simulink model "SolarMicroGrid"  (R2024b)
settings: Solver=VariableStepAuto  StartTime=0.0  StopTime=1  RelTol=1e-3
libraries: spsSeriesRLCBranchLib x9, spsMosfetLib x4, spsGroundLib x1, spsTriangleGeneratorLib x1, spsPVArrayLib x1, spsVoltageMeasurementLib x1, spsLinearTransformerLib x1, sps_lib x1
settings Model: Creator=Zidane Hadeed  LastModifiedBy=Zidane Hadeed

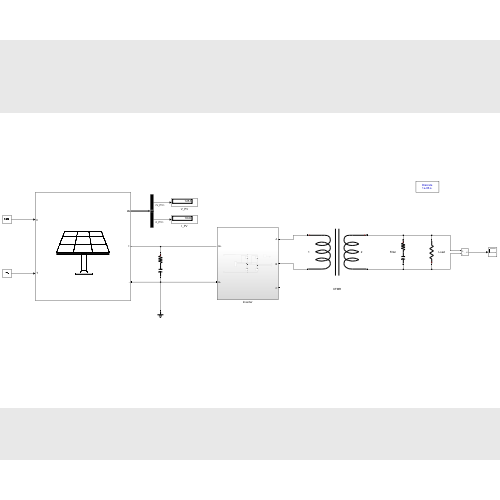
[thumbnail: Simulink's stored preview of the top-level diagram]
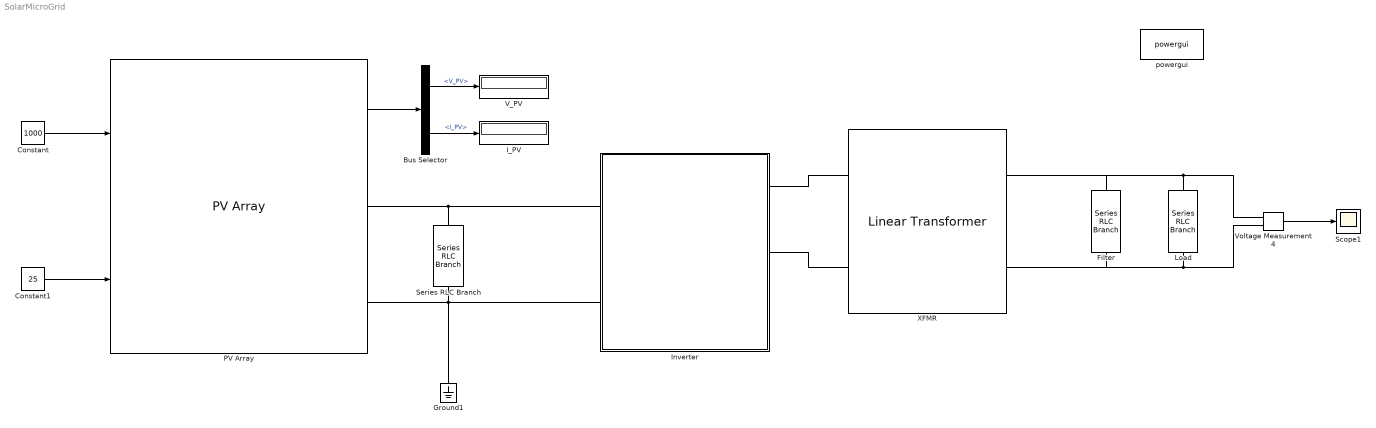
== system SolarMicroGrid ==
  Bus Selector : BusSelector  OutputSignals=V_PV,I_PV
  Constant : Constant  Value=1000
  Constant1 : Constant  Value=25
  Filter : spsSeriesRLCBranchLib/Series RLC Branch  LConnTagsString=__new0  RConnTagsString=__new0  BranchType=RC  Resistance=1e-3  Inductance=1e-3  SetiL0=off  InitialCurrent=0  Capacitance=1e-6  Setx0=off  InitialVoltage=0  Measurements=None
  Ground1 : spsGroundLib/Ground  LConnTagsString=a
  I_PV : Display
  Inverter : Subsystem
  Load : spsSeriesRLCBranchLib/Series RLC Branch  LConnTagsString=__new0  RConnTagsString=__new0  BranchType=R  Resistance=10e3  Inductance=1e-3  SetiL0=off  InitialCurrent=0  Capacitance=1e-6  Setx0=off  InitialVoltage=0  Measurements=None
  PV Array : spsPVArrayLib/PV Array  Npar=4  Nser=3  PlotType=array @ 25 deg.C & specified irradiances  S_vec="[ 1000  800  500 ]"  Temp_C_vec="[ 45 25  ]"  ModuleName=Aavid Solar ASMS-165P  PlotWhenSelected=off  Pm=164.85  Ncell=72  Voc=43.5  Isc=5.25  Vm=35  Im=4.71  beta_Voc_pc=-0.393  alpha_Isc_pc=0.03  beta_Voc=-0.17095  alpha_Isc=0.001575  IL=5.2764  I0=4.9875e-10  nI=1.0218  Rsh=125.0069  Rs=0.62818  RobustModel=off  RobustCellTemperature=313.3991  BAL=on  Tc=1e-6  Tfilter=5e-5
  Scope1 : Scope
  Series RLC Branch : spsSeriesRLCBranchLib/Series RLC Branch  LConnTagsString=__new0  RConnTagsString=__new0  BranchType=RC  Resistance=1e-2  Inductance=1e-3  SetiL0=off  InitialCurrent=0  Capacitance=4700e-6  Setx0=off  InitialVoltage=0  Measurements=None
  V_PV : Display
  Voltage Measurement4 : spsVoltageMeasurementLib/Voltage Measurement  PhasorSimulation=off  OutputType=Complex  PSBequivalent=0
  XFMR : spsLinearTransformerLib/Linear Transformer  UNITS=SI  NominalPower=[ 5e3 60 ]  winding1=[120 4.3218 0.45856]  winding2=[240 17.2872 1.83424]  ThreeWindings=off  winding3=[3.15e+05 0.7938 0.084225]  RmLm=[1.0804e+06 2866]  Measurements=All voltages and currents  DataType=on
  powergui : sps_lib/powergui  Priority=1  SimulationMode=Discrete  SampleTime=1e-6  frequency=60  Iterations=50  frequencyindice=0  Pbase=100e6  ErrMax=1e-4  UnitsV=kV  UnitsW=MW  buscounter=0  FunctionMessages=off  echomessages=off  EnableUseOfTLC=off  CurrentSourceSwitches=off  DisableSnubberDevices=off  DisableRonSwitches=off  DisableVfSwitches=off  DisplayEquations=off  AutomaticDiscreteSolvers=off  SolverType=Tustin/Backward Euler (TBE)  Interpol=off  ExternalGateDelay=off  methode=off  Ts=100  x0status=blocks  SPID=on  SwTol=0  HookPort=off  NonlinearTolerance=1e-4  nMaxIteration=100  ContinueOnMaxIteration=off  RestoreLinks=warning  ResistiveCurrentMeasurement=off  Frange=[0:2:500]  Ylog=off  Xlog=on  ShowGrid=off  save=off  variable=ZData  structure=0  ZoomFFT=off  StartTime=0.0  cycles=1  DisplayStyle=1  fundamental=60  FreqAxis=off  MaxFrequency=1000  frequencyindicesteady=1  RmsSteady=1  display=off
  wires:
  Voltage Measurement4/1 -> Scope1/1
  Constant1/1 -> PV Array/2
  PV Array/1 -> Bus Selector/1
  Constant/1 -> PV Array/1
  Bus Selector/1 -> V_PV/1  "<V_PV>"
  Bus Selector/2 -> I_PV/1  "<I_PV>"
  connections:
  Series RLC Branch/LConn1 -- Inverter/LConn1 -- PV Array/RConn1
  PV Array/RConn2 -- Ground1/LConn1 -- Series RLC Branch/RConn1 -- Inverter/LConn2
  Voltage Measurement4/LConn1 -- XFMR/RConn1 -- Filter/LConn1 -- Load/RConn1
  Load/LConn1 -- Filter/RConn1 -- XFMR/RConn2 -- Voltage Measurement4/LConn2
  XFMR/LConn1 -- Inverter/RConn1
  Inverter/RConn2 -- XFMR/LConn2

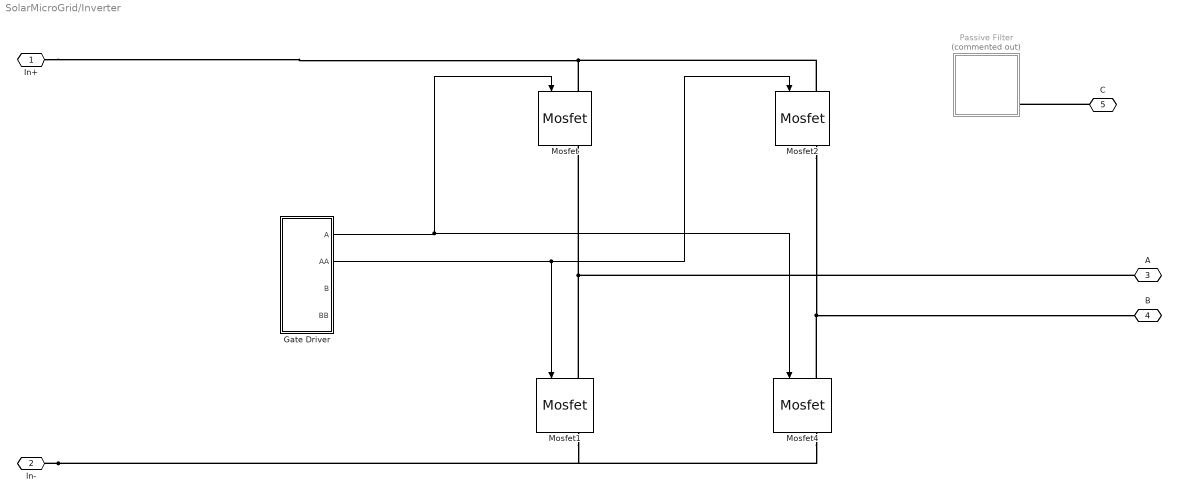
== system SolarMicroGrid/Inverter ==
  Gate Driver : Subsystem
  Mosfet{,1..2,4} (4 alike) : spsMosfetLib/Mosfet  Ron=0.1  Lon=0  Rd=0.01  Vfd=0  IC=0  Rs=1e5  Cs=inf  Measurements=on
  Passive Filter : Subsystem  Commented=on
      settings: PortSchema="{\"entries\":[{\"content\":{\"sides\":[{\"content\":{\"connectorIds\":[\"LConn1\",\"LConn2\",\"LConn3\"]},\"type\":\"ConnectorPlacement.EquallySpacedRectSide\",\"uuid\":\"62e55c9e-b411-4f10-a29f-aa0c5be36897\"},{\"content\":{\"connectorIds\":[\"RConn1\",\"RConn2\",\"RConn3\"],\"side\":\"RIGHT\"},\"type\":\"ConnectorPlacement.EquallySpacedRectSide\",\"uuid\":\"476f1a27-74f2-436a-8fc3-e2e5d83bb21b\"},{\"content\":{\"side\":\"TOP\"},\"type\":\"ConnectorPlacement.EquallySpacedRectSide\",\"uuid\":\"6a538d83-3a6b-4d9f-b9e9-43834189a8fd\"},{\"content\":{\"connectorIds\":[\"RConn4\"],\"side\":\"BOTTOM\"},\"type\":\"ConnectorPlacement.EquallySpacedRectSide\",\"uuid\":\"d798d2e6-cd10-429f-9f9b-8383104bce78\"}]},\"type\":\"ConnectorPlacement.EquallySpacedConnector\",\"uuid\":\"0b9f9509-cccf-4838-84a5-b9f3e67ee63a\"}],\"packageUris\":[\"http://schema.mathworks.com/mf0/Connector/R2020b\"],\"version\":\"1.0\"}"
  In+ : PMIOPort  Side=Left
  In- : PMIOPort  Port=2  Side=Left
  A : PMIOPort  Port=3  Side=Right
  B : PMIOPort  Port=4  Side=Right
  C : PMIOPort  Port=5  Side=Right
  wires:
  Gate Driver/1(A) -> Mosfet4/1, Mosfet/1
  Gate Driver/2(AA) -> Mosfet2/1, Mosfet1/1
  connections:
  In-/RConn1 -- Mosfet4/RConn1 -- Mosfet1/RConn1
  In+/RConn1 -- Mosfet2/LConn1 -- Mosfet/LConn1
  Mosfet1/LConn1 -- A/RConn1 -- Mosfet/RConn1
  Mosfet2/RConn1 -- Mosfet4/LConn1 -- B/RConn1
  C/RConn1 -- Passive Filter/RConn3

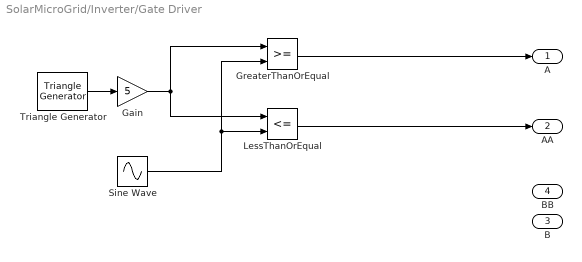
== system SolarMicroGrid/Inverter/Gate Driver ==
  Gain : Gain  Gain=5
  GreaterThanOrEqual : RelationalOperator  OutDataTypeStr=boolean  RndMeth=Simplest  InputSameDT=off
  LessThanOrEqual : RelationalOperator  Operator=<=  OutDataTypeStr=boolean  RndMeth=Simplest  InputSameDT=off
  Sine Wave : Sin  Amplitude=5  Frequency=100*pi  SampleTime=0
  Triangle Generator : spsTriangleGeneratorLib/Triangle Generator  Freq=300  Phase=0  Ts=0
  A : Outport
  AA : Outport  Port=2
  B : Outport  Port=3
  BB : Outport  Port=4
  wires:
  Sine Wave/1 -> GreaterThanOrEqual/2, LessThanOrEqual/2
  Triangle Generator/1 -> Gain/1
  Gain/1 -> LessThanOrEqual/1, GreaterThanOrEqual/1
  GreaterThanOrEqual/1 -> A/1
  LessThanOrEqual/1 -> AA/1

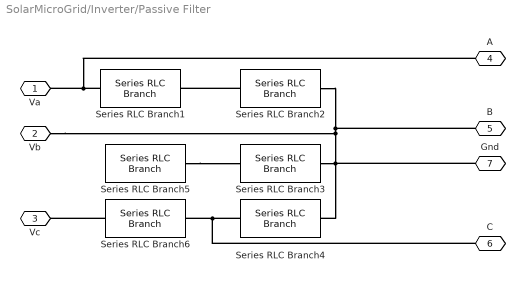
== system SolarMicroGrid/Inverter/Passive Filter ==
  Series RLC Branch1 : spsSeriesRLCBranchLib/Series RLC Branch  LConnTagsString=__new0  RConnTagsString=__new0  BranchType=L  Resistance=1  Inductance=100e-3  SetiL0=off  InitialCurrent=0  Capacitance=540e-3  Setx0=off  InitialVoltage=0  Measurements=None
  Series RLC Branch2 : spsSeriesRLCBranchLib/Series RLC Branch  LConnTagsString=__new0  RConnTagsString=__new0  BranchType=C  Resistance=1  Inductance=1e-3  SetiL0=off  InitialCurrent=0  Capacitance=0.1e-6  Setx0=off  InitialVoltage=0  Measurements=None
  Series RLC Branch3 : spsSeriesRLCBranchLib/Series RLC Branch  LConnTagsString=__new0  RConnTagsString=__new0  BranchType=C  Resistance=1  Inductance=1e-3  SetiL0=off  InitialCurrent=0  Capacitance=100e-6  Setx0=off  InitialVoltage=0  Measurements=None
  Series RLC Branch4 : spsSeriesRLCBranchLib/Series RLC Branch  LConnTagsString=__new0  RConnTagsString=__new0  BranchType=C  Resistance=1  Inductance=1e-3  SetiL0=off  InitialCurrent=0  Capacitance=100e-6  Setx0=off  InitialVoltage=0  Measurements=None
  Series RLC Branch5 : spsSeriesRLCBranchLib/Series RLC Branch  LConnTagsString=__new0  RConnTagsString=__new0  BranchType=L  Resistance=1  Inductance=100e-3  SetiL0=off  InitialCurrent=0  Capacitance=540e-3  Setx0=off  InitialVoltage=0  Measurements=None
  Series RLC Branch6 : spsSeriesRLCBranchLib/Series RLC Branch  LConnTagsString=__new0  RConnTagsString=__new0  BranchType=L  Resistance=1  Inductance=100e-3  SetiL0=off  InitialCurrent=0  Capacitance=540e-3  Setx0=off  InitialVoltage=0  Measurements=None
  Va : PMIOPort  Side=Left
  Vb : PMIOPort  Port=2  Side=Left
  Vc : PMIOPort  Port=3  Side=Left
  A : PMIOPort  Port=4  Side=Right
  B : PMIOPort  Port=5  Side=Right
  C : PMIOPort  Port=6  Side=Right
  Gnd : PMIOPort  Port=7  Side=Right
  connections:
  Series RLC Branch4/LConn1 -- C/RConn1 -- Series RLC Branch6/RConn1
  Series RLC Branch1/LConn1 -- A/RConn1 -- Va/RConn1
  Series RLC Branch2/RConn1 -- Vb/RConn1 -- Gnd/RConn1 -- Series RLC Branch3/RConn1 -- Series RLC Branch4/RConn1 -- B/RConn1
  Series RLC Branch2/LConn1 -- Series RLC Branch1/RConn1
  Series RLC Branch6/LConn1 -- Vc/RConn1
  Series RLC Branch5/RConn1 -- Series RLC Branch3/LConn1
